simulink library "flowVariants"  (R2017b)
settings: Solver=VariableStepAuto  StartTime=0.0  StopTime=10.0  RelTol=1e-3
undefined symbols (not defined in the file): env, p
settings Model: Creator=M.Cobb  LastModifiedBy=mitch
settings CodeAppCC: StateflowObjectComments=on

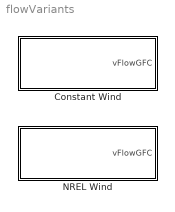
== system flowVariants ==
  Constant Wind : Subsystem
  NREL Wind : Subsystem

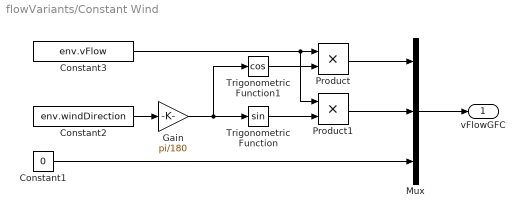
== system flowVariants/Constant Wind ==
  Constant1 : Constant  Value=0
  Constant2 : Constant  Value=env.windDirection
  Constant3 : Constant  Value=env.vFlow
  Gain : Gain  Gain=pi/180
  Mux : Mux  Inputs=3
  Product : Product
  Product1 : Product
  Trigonometric Function : Trigonometry
  Trigonometric Function1 : Trigonometry  Operator=cos
  vFlowGFC : Outport
  wires:
  Constant3/1 -> Product1/1, Product/1
  Gain/1 -> Trigonometric Function1/1, Trigonometric Function/1
  Product1/1 -> Mux/2
  Constant1/1 -> Mux/3
  Trigonometric Function/1 -> Product1/2
  Product/1 -> Mux/1
  Trigonometric Function1/1 -> Product/2
  Mux/1 -> vFlowGFC/1
  Constant2/1 -> Gain/1

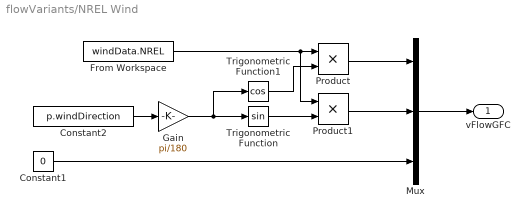
== system flowVariants/NREL Wind ==
  Constant1 : Constant  Value=0
  Constant2 : Constant  Value=p.windDirection
  From Workspace : FromWorkspace  VariableName=windData.NREL  SampleTime=0
  Gain : Gain  Gain=pi/180
  Mux : Mux  Inputs=3
  Product : Product
  Product1 : Product
  Trigonometric Function : Trigonometry
  Trigonometric Function1 : Trigonometry  Operator=cos
  vFlowGFC : Outport
  wires:
  Mux/1 -> vFlowGFC/1
  Product1/1 -> Mux/2
  Product/1 -> Mux/1
  Trigonometric Function/1 -> Product1/2
  Gain/1 -> Trigonometric Function1/1, Trigonometric Function/1
  Trigonometric Function1/1 -> Product/2
  Constant2/1 -> Gain/1
  Constant1/1 -> Mux/3
  From Workspace/1 -> Product1/1, Product/1
